simulink model "CP_ContrSys_NLin_b_n9329013"  (R2017b)
settings: Solver=ode4  StartTime=0.0  StopTime=10.0  FixedStep=0.02  RelTol=1e-3
values from neighbouring files (symbols this model uses):
  A_NL = A    [CP_ContrSys_Lin_a_Mainfile_n9329013.m]    (also in CP_ContrSys_Lin_b_Mainfile_n9329013.m)
  B_NL = B    [CP_ContrSys_Lin_a_Mainfile_n9329013.m]    (also in CP_ContrSys_Lin_b_Mainfile_n9329013.m)
  C_NL = CObs    [CP_ContrSys_Lin_a_Mainfile_n9329013.m]    (also in CP_ContrSys_Lin_b_Mainfile_n9329013.m)
  g = 9.81    [CP_ContrSys_Lin_a_Mainfile_n9329013.m]    (also in CP_ContrSys_Lin_b_Mainfile_n9329013.m; MainFile_9329013.m; MainFile_Linearised_a_9329013.m; MainFile_Linearised_b_9329013.m)
  initial_cond = [0.2,20*pi/180, 0,0]'    [CP_ContrSys_Lin_a_Mainfile_n9329013.m]    (also in CP_ContrSys_Lin_b_Mainfile_n9329013.m = [0.2,200*pi/180, 0,0]')
  K_SF = Ka    [CP_ContrSys_Lin_a_Mainfile_n9329013.m]    (also in CP_ContrSys_Lin_b_Mainfile_n9329013.m = Kb)
  l = 0.2    [CP_ContrSys_Lin_a_Mainfile_n9329013.m]    (also in CP_ContrSys_Lin_b_Mainfile_n9329013.m; MainFile_9329013.m; MainFile_Linearised_a_9329013.m; MainFile_Linearised_b_9329013.m)
  L_NL = La    [CP_ContrSys_Lin_a_Mainfile_n9329013.m]    (also in CP_ContrSys_Lin_b_Mainfile_n9329013.m = Lb)
  m = 0.15    [CP_ContrSys_Lin_a_Mainfile_n9329013.m]    (also in CP_ContrSys_Lin_b_Mainfile_n9329013.m; MainFile_9329013.m; MainFile_Linearised_a_9329013.m; MainFile_Linearised_b_9329013.m)
  Mc = 0.4    [CP_ContrSys_Lin_a_Mainfile_n9329013.m]    (also in CP_ContrSys_Lin_b_Mainfile_n9329013.m; MainFile_9329013.m; MainFile_Linearised_a_9329013.m; MainFile_Linearised_b_9329013.m)
  x1_bar = 0    [CP_ContrSys_Lin_a_Mainfile_n9329013.m]    (also in CP_ContrSys_Lin_b_Mainfile_n9329013.m)
  x2_bar = 0    [CP_ContrSys_Lin_a_Mainfile_n9329013.m]    (also in CP_ContrSys_Lin_b_Mainfile_n9329013.m = 3.14159265359)
  x3_bar = 0    [CP_ContrSys_Lin_a_Mainfile_n9329013.m]    (also in CP_ContrSys_Lin_b_Mainfile_n9329013.m)
  x4_bar = 0    [CP_ContrSys_Lin_a_Mainfile_n9329013.m]    (also in CP_ContrSys_Lin_b_Mainfile_n9329013.m)
settings Model: Creator=Koh Kim Hai  LastModifiedBy=Koh Kim Hai
settings DataIOCC: TimeSaveName=t

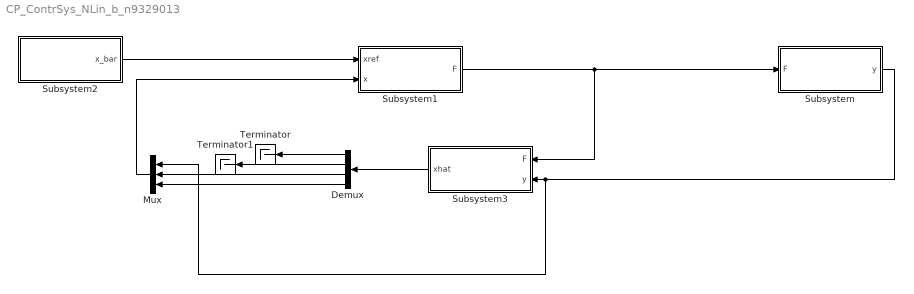
== system CP_ContrSys_NLin_b_n9329013 ==
  Demux : Demux
  Mux : Mux  Inputs=3
  Subsystem : Subsystem
  Subsystem1 : Subsystem
  Subsystem2 : Subsystem
  Subsystem3 : Subsystem
  Terminator : Terminator
  Terminator1 : Terminator
  wires:
  Subsystem2/1(x_bar) -> Subsystem1/1(xref)
  Subsystem1/1(F) -> Subsystem3/1(F), Subsystem/1(F)
  Subsystem/1(y) -> Mux/1, Subsystem3/2(y)
  Subsystem3/1(xhat) -> Demux/1
  Demux/1 -> Terminator/1
  Demux/2 -> Terminator1/1
  Demux/3 -> Mux/2
  Demux/4 -> Mux/3
  Mux/1 -> Subsystem1/2(x)

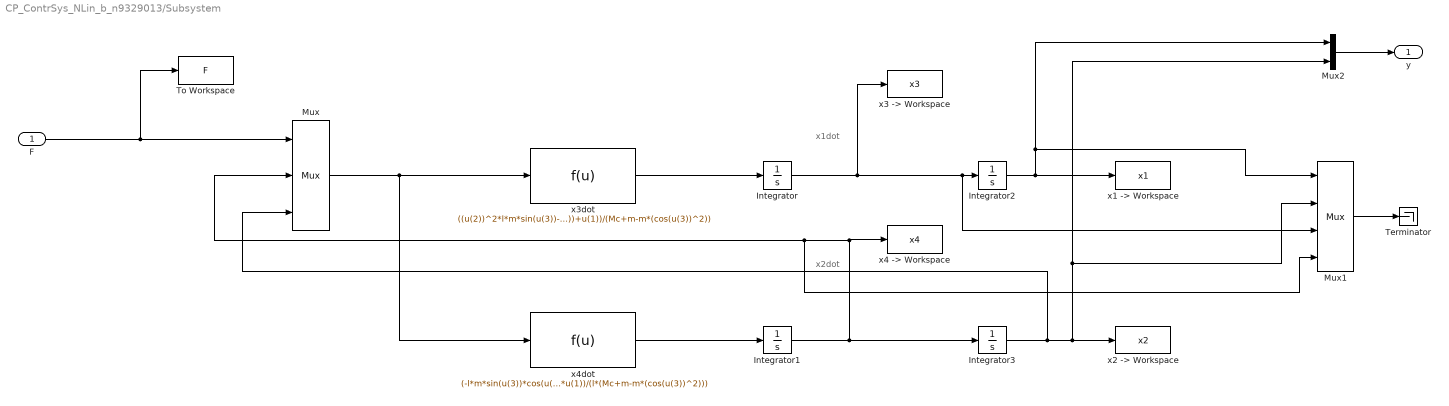
== system CP_ContrSys_NLin_b_n9329013/Subsystem ==
  note: x1dot
  note: x2dot
  F : Inport
  Integrator : Integrator  InitialCondition=initial_cond(3)
  Integrator1 : Integrator  InitialCondition=initial_cond(4)
  Integrator2 : Integrator  InitialCondition=initial_cond(1)
  Integrator3 : Integrator  InitialCondition=200*pi/180
  Mux : Mux  Inputs=3
  Mux1 : Mux
  Mux2 : Mux  Inputs=2
  Terminator : Terminator
  To Workspace : ToWorkspace  VariableName=F  SampleTime=-1
  "x1 -> Workspace" : ToWorkspace  VariableName=x1  SampleTime=-1
  "x2 -> Workspace" : ToWorkspace  VariableName=x2  SampleTime=-1
  "x3 -> Workspace" : ToWorkspace  VariableName=x3  SampleTime=-1
  x3dot : Fcn  Expr=((u(2))^2*l*m*sin(u(3))-g*m*sin(u(3))*cos(u(3))+u(1))/(Mc+m-m*(cos(u(3))^2))
  "x4 -> Workspace" : ToWorkspace  VariableName=x4  SampleTime=-1
  x4dot : Fcn  Expr=(-l*m*sin(u(3))*cos(u(3))*(u(2))^2+g*(Mc+m)*sin(u(3))-cos(u(3))*u(1))/(l*(Mc+m-m*(cos(u(3))^2)))
  y : Outport
  wires:
  Integrator3/1 -> Mux/3, Mux2/2, Mux1/2, "x2 -> Workspace"/1
  Integrator/1 -> "x3 -> Workspace"/1, Mux1/3, Integrator2/1
  F/1 -> To Workspace/1, Mux/1
  Integrator1/1 -> Mux1/4, Mux/2, "x4 -> Workspace"/1, Integrator3/1
  Mux/1 -> x4dot/1, x3dot/1
  x3dot/1 -> Integrator/1
  x4dot/1 -> Integrator1/1
  Mux1/1 -> Terminator/1
  Integrator2/1 -> Mux2/1, Mux1/1, "x1 -> Workspace"/1
  Mux2/1 -> y/1

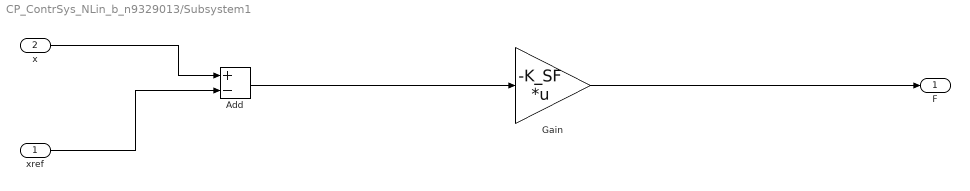
== system CP_ContrSys_NLin_b_n9329013/Subsystem1 ==
  xref : Inport
  x : Inport  Port=2
  Add : Sum  Inputs=+-
  Gain : Gain  Gain=-K_SF  Multiplication=Matrix(K*u)
  F : Outport
  wires:
  Gain/1 -> F/1
  xref/1 -> Add/2
  x/1 -> Add/1
  Add/1 -> Gain/1

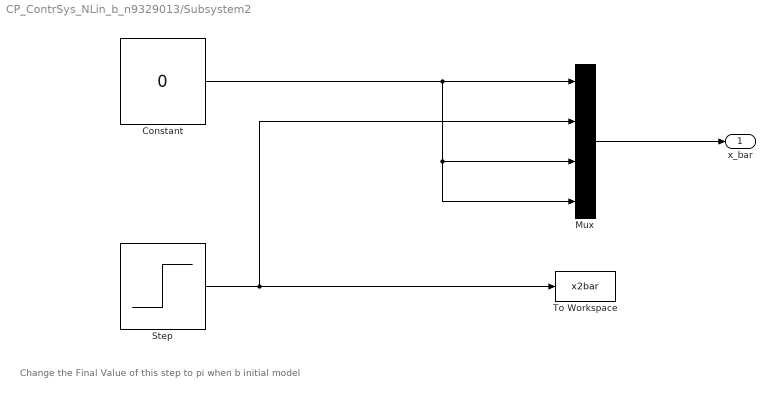
== system CP_ContrSys_NLin_b_n9329013/Subsystem2 ==
  note: Change the Final Value of this step to pi when b initial model
  Constant : Constant  Value=0
  Mux : Mux
  Step : Step  Time=0  After=pi  SampleTime=0
  To Workspace : ToWorkspace  VariableName=x2bar  SampleTime=-1
  x_bar : Outport
  wires:
  Mux/1 -> x_bar/1
  Constant/1 -> Mux/4, Mux/3, Mux/1
  Step/1 -> To Workspace/1, Mux/2

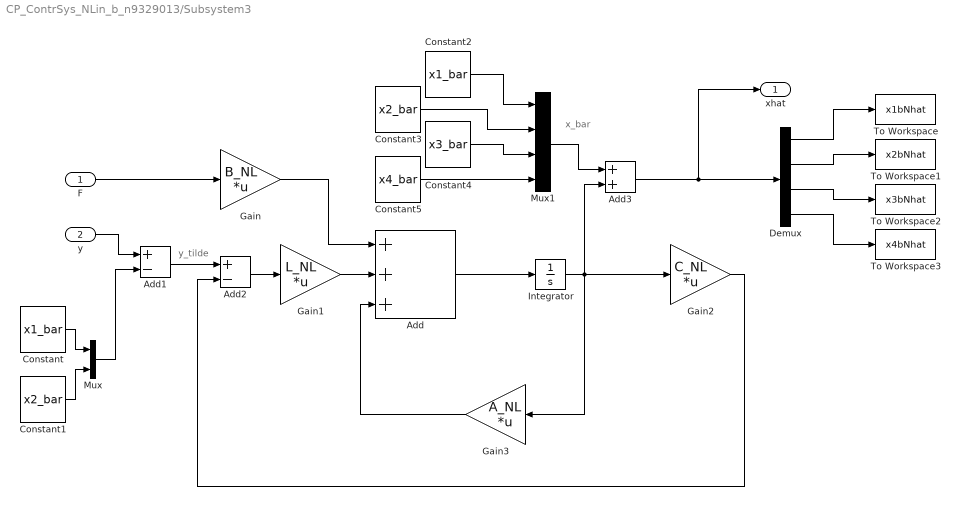
== system CP_ContrSys_NLin_b_n9329013/Subsystem3 ==
  note: x_bar
  note: y_tilde
  F : Inport
  y : Inport  Port=2
  Add : Sum  Inputs=+++
  Add1 : Sum  Inputs=+-
  Add2 : Sum  Inputs=+-
  Add3 : Sum  Inputs=2
  Constant : Constant  Value=x1_bar
  Constant1 : Constant  Value=x2_bar
  Constant2 : Constant  Value=x1_bar
  Constant3 : Constant  Value=x2_bar
  Constant4 : Constant  Value=x3_bar
  Constant5 : Constant  Value=x4_bar
  Demux : Demux
  Gain : Gain  Gain=B_NL  Multiplication=Matrix(K*u)
  Gain1 : Gain  Gain=L_NL  Multiplication=Matrix(K*u)
  Gain2 : Gain  Gain=C_NL  Multiplication=Matrix(K*u)
  Gain3 : Gain  Gain=A_NL  Multiplication=Matrix(K*u)
  Integrator : Integrator
  Mux : Mux  Inputs=2
  Mux1 : Mux
  To Workspace : ToWorkspace  VariableName=x1bNhat  SampleTime=-1
  To Workspace1 : ToWorkspace  VariableName=x2bNhat  SampleTime=-1
  To Workspace2 : ToWorkspace  VariableName=x3bNhat  SampleTime=-1
  To Workspace3 : ToWorkspace  VariableName=x4bNhat  SampleTime=-1
  xhat : Outport
  wires:
  F/1 -> Gain/1
  Gain1/1 -> Add/2
  Gain/1 -> Add/1
  Gain3/1 -> Add/3
  Add/1 -> Integrator/1
  y/1 -> Add1/1
  Integrator/1 -> Gain3/1, Gain2/1, Add3/2
  Demux/1 -> To Workspace/1
  Demux/2 -> To Workspace1/1
  Demux/3 -> To Workspace2/1
  Demux/4 -> To Workspace3/1
  Constant/1 -> Mux/1
  Constant1/1 -> Mux/2
  Mux/1 -> Add1/2
  Add2/1 -> Gain1/1
  Add1/1 -> Add2/1
  Gain2/1 -> Add2/2
  Constant4/1 -> Mux1/3
  Constant2/1 -> Mux1/1
  Constant5/1 -> Mux1/4
  Mux1/1 -> Add3/1
  Add3/1 -> Demux/1, xhat/1
  Constant3/1 -> Mux1/2
